simulink subsystem "Day3_Scenario_1"  (R2024a)
settings: Solver=VariableStepAuto  StartTime=0.0  StopTime=10.0  RelTol=1e-3
undefined symbols (not defined in the file): left_first_line_point_x, right_first_line_point_x
libraries: CarMaker4SL x6, slpidlib x1
settings Model: Creator=junhyung.cha  LastModifiedBy=hajin

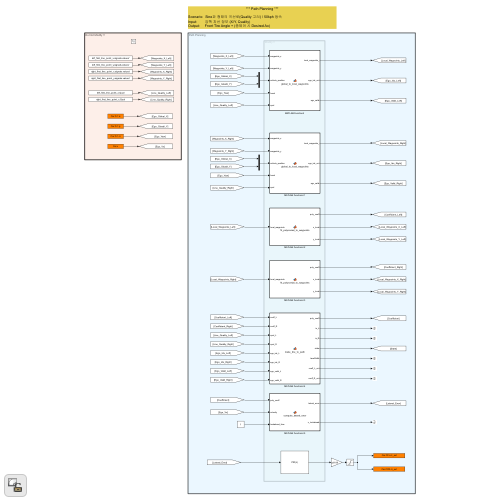
[thumbnail: Simulink's stored preview of the top-level diagram]
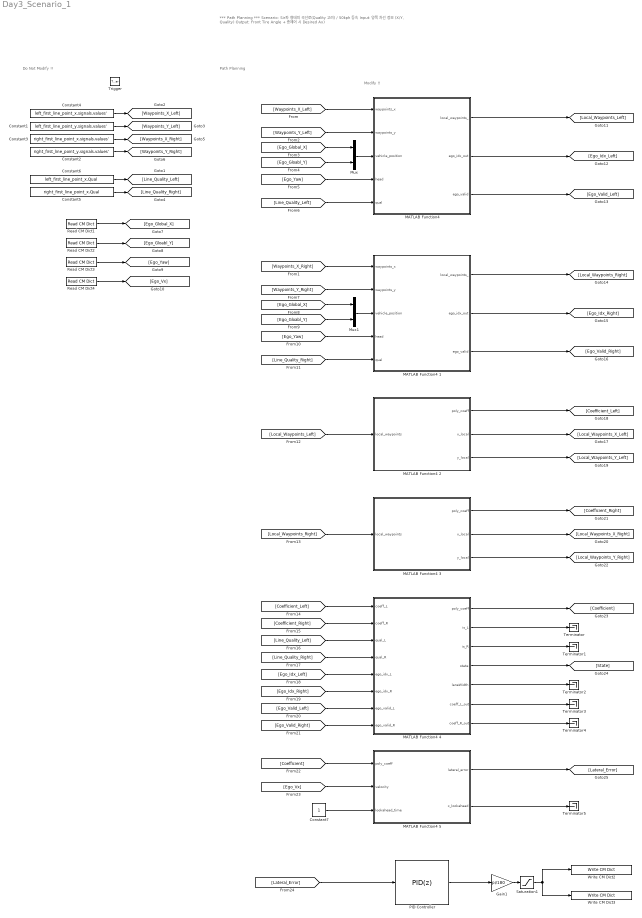
== system Day3_Scenario_1 ==
  note: Path Planning
  note: Do Not Modify !!
  note: Modify !!
  note: *** Path Planning ***
      |
      | Scenario: Sine파 형태의 곡선로(Quality 고려) / 50kph 등속
      | Input: 양쪽 차선 정보 (X/Y, Quality)
      | Output: Front Tire Angle + (종제어 시 Desired Ax)
  Trigger : TriggerPort  TriggerType=function-call  VariantControl=(inherit)
  Constant1 : Constant  Value=left_first_line_point_y.signals.values'
  Constant2 : Constant  Value=right_first_line_point_y.signals.values'
  Constant3 : Constant  Value=right_first_line_point_x.signals.values'
  Constant4 : Constant  Value=left_first_line_point_x.signals.values'
  Constant5 : Constant  Value=right_first_line_point_x.Qual
  Constant6 : Constant  Value=left_first_line_point_x.Qual
  Constant7 : Constant
  Gain1 : Gain  Gain=pi/180
  "MATLAB Function4 " : MATLAB Function  TreatAsAtomicUnit=on
  MATLAB Function4 1 : MATLAB Function  TreatAsAtomicUnit=on
  MATLAB Function4 2 : MATLAB Function  TreatAsAtomicUnit=on
  MATLAB Function4 3 : MATLAB Function  TreatAsAtomicUnit=on
  MATLAB Function4 4 : MATLAB Function  TreatAsAtomicUnit=on
  MATLAB Function4 5 : MATLAB Function  TreatAsAtomicUnit=on
  Mux : Mux  Inputs=2
  Mux1 : Mux  Inputs=2
  PID Controller : slpidlib/PID Controller  Controller=PID  Form=Parallel  TimeDomain=Discrete-time  UseExternalTs=off  SampleTime=-1  IntegratorMethod=Forward Euler  FilterMethod=Forward Euler  ControllerParametersSource=internal  P=3  I=0  UseKiTs=off  D=0.8  UseExternalDerivativeSource=off  N=100  UseFilter=on  TunerSelectOption=Transfer Function Based (PID Tuner App)  InitialConditionSource=internal  InitialConditionForIntegrator=0  InitialConditionForFilter=0  DifferentiatorICPrevScaledInput=0  ExternalReset=none  TrackingMode=off  Kt=1  LimitOutput=off  SatLimitsSource=internal  UpperSaturationLimit=inf  LowerSaturationLimit=-inf  LinearizeAsGain=on  AntiWindupMode=none  Kb=1  LimitIntegrator=off  UpperIntegratorSaturationLimit=inf  LowerIntegratorSaturationLimit=-inf  POutMin=[]  POutMax=[]  IOutMin=[]  IOutMax=[]  DOutMin=[]  DOutMax=[]  NOutMin=[]  NOutMax=[]  SumOutMin=[]  SumOutMax=[]  SaturationOutMin=[]  SaturationOutMax=[]  PParamMin=[]  PParamMax=[]  IParamMin=[]  IParamMax=[]  DParamMin=[]  DParamMax=[]  NParamMin=[]  NParamMax=[]  KbParamMin=[]  KbParamMax=[]  KtParamMin=[]  KtParamMax=[]  KbOutMin=[]  KbOutMax=[]  KtOutMin=[]  KtOutMax=[]  IntegratorOutMin=[]  IntegratorOutMax=[]  FilterOutMin=[]  FilterOutMax=[]  SumI1OutMin=[]  SumI1OutMax=[]  SumI2OutMin=[]  SumI2OutMax=[]  SumI3OutMin=[]  SumI3OutMax=[]  SumI4OutMin=[]  SumI4OutMax=[]  SumDOutMin=[]  SumDOutMax=[]  DifferentiatorOutMin=[]  DifferentiatorOutMax=[]  FilterDiffOutCoefMin=[]  FilterDiffOutCoefMax=[]  ReciprocalOutMin=[]  ReciprocalOutMax=[]  SumDenOutMin=[]  SumDenOutMax=[]  SumNumOutMin=[]  SumNumOutMax=[]  DivideOutMin=[]  DivideOutMax=[]  UdiffTsProdOutMin=[]  UdiffTsProdOutMax=[]  NTsProdOutMin=[]  NTsProdOutMax=[]  UintegralTsProdOutMin=[]  UintegralTsProdOutMax=[]  UngainTsProdOutMin=[]  UngainTsProdOutMax=[]  ClampingZeroOutDataTypeStr=Inherit: Inherit via back propagation  ClampingZeroOutMin=[]  ClampingZeroOutMax=[]  FilterDenConstantOutDataTypeStr=Inherit: Inherit via back propagation  FilterDenConstantOutMin=[]  FilterDenConstantOutMax=[]  PCopyOutDataTypeStr=Inherit: Inherit via back propagation  PCopyOutMin=[]  PCopyOutMax=[]  NCopyOutDataTypeStr=Inherit: Inherit via back propagation  NCopyOutMin=[]  NCopyOutMax=[]  IntegratorContinuousStateAttributes=''  IntegratorStateMustResolveToSignalObject=off  IntegratorRTWStateStorageClass=Auto  FilterContinuousStateAttributes=''  FilterStateMustResolveToSignalObject=off  FilterRTWStateStorageClass=Auto  ParallelPVariant=InternalParameters  IdealPVariant=Disabled  IVariant=InternalParameters  DVariant=InternalParameters  IntegratorVariant=Discrete  SatVariant=Disabled  AWVariant=Passthrough  PCopyVariant=Disabled  TRVariant=Disabled  FdbkBlocksVariant=Forward  IdealPFdbkVariant=Disabled  SatFdbkVariant=Disabled  DerivativeFilterVariant=ForwardEulerFilter  NVariant=InternalParameters  NCopyVariant=Disabled  FilterICVariant=InternalICsFilter  IntegratorICVariant=InternalICs  ExternalResetVariant=Disabled  TRSumVariant=Passthrough  SumFdbkVariant=Disabled  SumVariant=Sum_PID  TsampFilterVariant=InternalTs  TsampNgainVariant=Passthrough  TsampIntegralVariant=Disabled_SignalSpec  ExternalSaturationOutDataTypeStr=Inherit: Same as second input  DerivativeSourceVariant=ErrorSignal
  Read CM Dict1 : CarMaker4SL/Read CM Dict  xname=Car.Fr1.tx  xsync=off  xstime=Inherited
  Read CM Dict2 : CarMaker4SL/Read CM Dict  xname=Car.Fr1.ty  xsync=off  xstime=Inherited
  Read CM Dict3 : CarMaker4SL/Read CM Dict  xname=Car.Fr1.rz  xsync=off  xstime=Inherited
  Read CM Dict4 : CarMaker4SL/Read CM Dict  xname=Car.v  xsync=off  xstime=Inherited
  Saturation1 : Saturate  UpperLimit=2  LowerLimit=-2
  Terminator{,1..5} (6 alike) : Terminator
  Write CM Dict2 : CarMaker4SL/Write CM Dict  xname=Car.CFL.rz_ext  xsync=off
  Write CM Dict3 : CarMaker4SL/Write CM Dict  xname=Car.CFR.rz_ext  xsync=off
  wires:
  Constant4/1 -> [Waypoints_X_Left]
  Constant1/1 -> [Waypoints_Y_Left]
  Constant2/1 -> [Waypoints_Y_Right]
  Constant3/1 -> [Waypoints_X_Right]
  [Waypoints_X_Left] -> "MATLAB Function4 "/1(waypoints_x)
  [Waypoints_Y_Left] -> "MATLAB Function4 "/2(waypoints_y)
  Mux/1 -> "MATLAB Function4 "/3(vehicle_position)
  [Ego_Global_X] -> Mux/1
  Read CM Dict2/1 -> [Ego_Gloabl_Y]
  Read CM Dict1/1 -> [Ego_Global_X]
  [Ego_Gloabl_Y] -> Mux/2
  Read CM Dict3/1 -> [Ego_Yaw]
  [Ego_Yaw] -> "MATLAB Function4 "/4(head)
  Constant5/1 -> [Line_Quality_Right]
  Constant6/1 -> [Line_Quality_Left]
  [Line_Quality_Left] -> "MATLAB Function4 "/5(qual)
  [Line_Quality_Right] -> MATLAB Function4 1/5(qual)
  [Ego_Yaw] -> MATLAB Function4 1/4(head)
  [Ego_Gloabl_Y] -> Mux1/2
  [Ego_Global_X] -> Mux1/1
  [Waypoints_Y_Right] -> MATLAB Function4 1/2(waypoints_y)
  [Waypoints_X_Right] -> MATLAB Function4 1/1(waypoints_x)
  Mux1/1 -> MATLAB Function4 1/3(vehicle_position)
  "MATLAB Function4 "/3(ego_valid) -> [Ego_Valid_Left]
  "MATLAB Function4 "/2(ego_idx_out) -> [Ego_Idx_Left]
  "MATLAB Function4 "/1(local_waypoints_) -> [Local_Waypoints_Left]
  MATLAB Function4 1/1(local_waypoints_) -> [Local_Waypoints_Right]
  MATLAB Function4 1/2(ego_idx_out) -> [Ego_Idx_Right]
  MATLAB Function4 1/3(ego_valid) -> [Ego_Valid_Right]
  [Local_Waypoints_Left] -> MATLAB Function4 2/1(local_waypoints)
  [Local_Waypoints_Right] -> MATLAB Function4 3/1(local_waypoints)
  MATLAB Function4 2/1(poly_coeff) -> [Coefficient_Left]
  MATLAB Function4 2/2(x_local) -> [Local_Waypoints_X_Left]
  MATLAB Function4 2/3(y_local) -> [Local_Waypoints_Y_Left]
  MATLAB Function4 3/3(y_local) -> [Local_Waypoints_Y_Right]
  MATLAB Function4 3/2(x_local) -> [Local_Waypoints_X_Right]
  MATLAB Function4 3/1(poly_coeff) -> [Coefficient_Right]
  [Coefficient_Left] -> MATLAB Function4 4/1(coeff_L)
  [Coefficient_Right] -> MATLAB Function4 4/2(coeff_R)
  [Line_Quality_Left] -> MATLAB Function4 4/3(qual_L)
  [Line_Quality_Right] -> MATLAB Function4 4/4(qual_R)
  [Ego_Idx_Left] -> MATLAB Function4 4/5(ego_idx_L)
  [Ego_Idx_Right] -> MATLAB Function4 4/6(ego_idx_R)
  [Ego_Valid_Left] -> MATLAB Function4 4/7(ego_valid_L)
  [Ego_Valid_Right] -> MATLAB Function4 4/8(ego_valid_R)
  MATLAB Function4 4/1(poly_coeff) -> [Coefficient]
  MATLAB Function4 4/4(state) -> [State]
  MATLAB Function4 4/2(is_L) -> Terminator/1
  MATLAB Function4 4/3(is_R) -> Terminator1/1
  MATLAB Function4 4/6(coeff_L_out) -> Terminator3/1
  MATLAB Function4 4/5(laneWidth) -> Terminator2/1
  MATLAB Function4 4/7(coeff_R_out) -> Terminator4/1
  [Coefficient] -> MATLAB Function4 5/1(poly_coeff)
  Read CM Dict4/1 -> [Ego_Vx]
  [Ego_Vx] -> MATLAB Function4 5/2(velocity)
  Constant7/1 -> MATLAB Function4 5/3(lookahead_time)
  Saturation1/1 -> Write CM Dict3/1, Write CM Dict2/1
  Gain1/1 -> Saturation1/1
  MATLAB Function4 5/1(lateral_error) -> [Lateral_Error]
  MATLAB Function4 5/2(x_lookahead) -> Terminator5/1
  [Lateral_Error] -> PID Controller/1
  PID Controller/1 -> Gain1/1

== matlab function Day3_Scenario_1/MATLAB Function4  ==
  settings: sampleTime=0.1
  data: waypoints_x input; waypoints_y input; local_waypoints_ output; vehicle_position input; head input; qual input; ego_idx_out output; ego_valid output
function [local_waypoints_, ego_idx_out, ego_valid] = global_to_local_waypoints(waypoints_x, waypoints_y, vehicle_position, head, qual)
% 전역 좌표계 waypoint를 ego 차량 기준 local 좌표계로 변환하는 함수
%
% 입력:
%   waypoints_x       : 전역 waypoint X 좌표 배열
%   waypoints_y       : 전역 waypoint Y 좌표 배열
%   vehicle_position  : ego 차량 위치 [X, Y]
%   head              : ego 차량 yaw angle [rad]
%   qual              : 차선 quality 값
%
% 출력:
%   local_waypoints_  : ego 기준 local waypoint [x_local, y_local]
%   ego_idx_out       : ego 앞쪽에서 처음으로 유효한 waypoint의 원본 index
%   ego_valid         : 경로 생성에 사용할 수 있는 waypoint가 충분한지 여부

% waypoint 개수
N = length(waypoints_x);

% 출력 초기화
% NaN으로 채워두면 유효하지 않은 점은 이후 polyfit에서 제외하기 쉬움
local_waypoints_ = NaN(N, 2);
ego_idx_out = 0;
ego_valid = false;

% ego 차량의 전역 위치
ego_x = vehicle_position(1);
ego_y = vehicle_position(2);

% yaw 회전 변환을 위한 값
c = cos(head);
s = sin(head);

% 유효한 local waypoint 개수
valid_count = 0;

% 전방 첫 번째 유효 waypoint의 원본 index 저장용
first_valid_idx = 0;

for i = 1:N

    % quality가 scalar로 들어오는 경우와 배열로 들어오는 경우 모두 처리
    if length(qual) == 1
        point_valid = qual > 0.5;
    else
        point_valid = qual(i) > 0.5;
    end

    % quality가 유효한 점만 사용
    if point_valid

        % ego 위치 기준으로 평행이동
        dx = waypoints_x(i) - ego_x;
        dy = waypoints_y(i) - ego_y;

        % global 좌표계에서 local 좌표계로 회전 변환
        % ego 차량 진행 방향이 local x축
        x_local =  c * dx + s * dy;
        y_local = -s * dx + c * dy;

        % 차량 앞쪽에 있는 waypoint만 사용
        if x_local >= 0
            valid_count = valid_count + 1;

            local_waypoints_(valid_count, 1) = x_local;
            local_waypoints_(valid_count, 2) = y_local;

            % 처음 발견한 전방 유효 waypoint index 저장
            if first_valid_idx == 0
                first_valid_idx = i;
            end
        end
    end
end

% ego 앞쪽에서 처음으로 유효한 waypoint의 원본 index
ego_idx_out = first_valid_idx;

% 3차 다항식 피팅을 하려면 최소 4개의 점이 필요
if valid_count >= 4
    ego_valid = true;
else
    ego_valid = false;
end

end

== matlab function Day3_Scenario_1/MATLAB Function4 1 ==
  settings: sampleTime=0.1
  data: waypoints_x input; waypoints_y input; local_waypoints_ output; vehicle_position input; head input; qual input; ego_idx_out output; ego_valid output
function [local_waypoints_, ego_idx_out, ego_valid] = global_to_local_waypoints(waypoints_x, waypoints_y, vehicle_position, head, qual)
% 전역 좌표계의 waypoint를 ego 차량 기준 local 좌표계로 변환하는 함수
%
% 입력:
%   waypoints_x      : 전역 좌표계 waypoint X 배열
%   waypoints_y      : 전역 좌표계 waypoint Y 배열
%   vehicle_position : ego 차량의 전역 위치 [X, Y]
%   head             : ego 차량의 yaw angle [rad]
%   qual             : 차선 품질 값
%
% 출력:
%   local_waypoints_ : ego 기준 local waypoint [x_local, y_local]
%   ego_idx_out      : ego 앞쪽에서 처음 발견된 유효 waypoint index
%   ego_valid        : 경로 생성에 사용할 수 있는 waypoint가 충분한지 여부

% 입력 waypoint를 column vector로 변환
waypoints_x = waypoints_x(:);
waypoints_y = waypoints_y(:);

% waypoint 개수 확인
N = length(waypoints_x);

% 출력 초기화
% 유효하지 않은 waypoint는 NaN으로 남김
local_waypoints_ = NaN(N, 2);
ego_idx_out = 0;
ego_valid = false;

% ego 차량의 전역 위치
ego_x = vehicle_position(1);
ego_y = vehicle_position(2);

% heading angle에 대한 삼각함수 계산
c = cos(head);
s = sin(head);

% 유효한 전방 waypoint 개수
valid_count = 0;

% quality 기준값
quality_threshold = 0.5;

for i = 1:N

    % quality가 scalar로 들어오는 경우
    if length(qual) == 1
        point_valid = qual > quality_threshold;

    % quality가 waypoint별 배열로 들어오는 경우
    else
        point_valid = qual(i) > quality_threshold;
    end

    % quality가 좋지 않으면 해당 waypoint는 사용하지 않음
    if point_valid

        % ego 차량 위치 기준으로 평행 이동
        dx = waypoints_x(i) - ego_x;
        dy = waypoints_y(i) - ego_y;

        % global 좌표계에서 ego 기준 local 좌표계로 회전 변환
        % local x축 : 차량 진행 방향
        % local y축 : 차량 좌측 방향
        x_local =  c * dx + s * dy;
        y_local = -s * dx + c * dy;

        % 차량 앞쪽에 있는 waypoint만 사용
        if x_local >= 0

            valid_count = valid_count + 1;

            % local waypoint 저장
            local_waypoints_(valid_count, 1) = x_local;
            local_waypoints_(valid_count, 2) = y_local;

            % ego 앞쪽에서 처음 발견된 waypoint의 원본 index 저장
            if ego_idx_out == 0
                ego_idx_out = i;
            end
        end
    end
end

% 3차 다항식 fitting을 위해서는 최소 4개의 점이 필요
if valid_count >= 4
    ego_valid = true;
else
    ego_valid = false;
end

end

== matlab function Day3_Scenario_1/MATLAB Function4 2 ==
  settings: sampleTime=0.1
  data: local_waypoints input; poly_coeff output; x_local output; y_local output
function [poly_coeff, x_local, y_local] = fit_polynomial_to_waypoints(local_waypoints)
% local waypoint들을 이용해 3차 다항식 계수를 계산하는 함수
% Simulink MATLAB Function 블록에서 가변 크기 오류를 피하기 위한 고정 크기 코드

% 입력 waypoint 개수
N = size(local_waypoints, 1);

% 출력 초기화
% poly_coeff는 항상 [4x1] 고정
poly_coeff = zeros(4, 1);

% x_local, y_local은 입력 waypoint 개수만큼 고정
x_local = zeros(N, 1);
y_local = zeros(N, 1);

% 다항식 피팅에 사용할 최대 점 개수
% 너무 많은 점을 모두 쓰지 않고 앞쪽 유효 점 일부만 사용
max_fit_num = 20;

% 피팅용 배열 고정 크기 선언
x_fit = zeros(max_fit_num, 1);
y_fit = zeros(max_fit_num, 1);

valid_count = 0;

% 유효한 waypoint 수집
for i = 1:N
    x = local_waypoints(i, 1);
    y = local_waypoints(i, 2);

    % NaN이 아니고 차량 앞쪽에 있는 점만 사용
    if isfinite(x) && isfinite(y) && x >= 0

        % 출력 확인용 local 좌표 저장
        x_local(i) = x;
        y_local(i) = y;

        % 피팅에는 최대 max_fit_num개만 사용
        if valid_count < max_fit_num
            valid_count = valid_count + 1;
            x_fit(valid_count) = x;
            y_fit(valid_count) = y;
        end
    end
end

% 유효한 점이 4개 이상이면 3차 다항식 피팅
if valid_count >= 4

    % 고정 크기 행렬 사용
    A = zeros(max_fit_num, 4);
    b = zeros(max_fit_num, 1);

    for i = 1:max_fit_num
        x = x_fit(i);

        A(i, 1) = x^3;
        A(i, 2) = x^2;
        A(i, 3) = x;
        A(i, 4) = 1;

        b(i) = y_fit(i);
    end

    % 최소자승법
    % 결과는 항상 [4x1]
    coeff_temp = A \ b;

    poly_coeff(1) = coeff_temp(1);
    poly_coeff(2) = coeff_temp(2);
    poly_coeff(3) = coeff_temp(3);
    poly_coeff(4) = coeff_temp(4);

% 유효한 점이 2~3개면 1차 직선으로 대체
elseif valid_count >= 2

    A_line = zeros(max_fit_num, 2);
    b_line = zeros(max_fit_num, 1);

    for i = 1:max_fit_num
        x = x_fit(i);

        A_line(i, 1) = x;
        A_line(i, 2) = 1;

        b_line(i) = y_fit(i);
    end

    line_coeff = A_line \ b_line;

    % 3차 계수 형태로 고정 출력
    % y = 0*x^3 + 0*x^2 + m*x + b
    poly_coeff(1) = 0;
    poly_coeff(2) = 0;
    poly_coeff(3) = line_coeff(1);
    poly_coeff(4) = line_coeff(2);

else

    % 유효한 점이 부족하면 직진 경로
    poly_coeff(1) = 0;
    poly_coeff(2) = 0;
    poly_coeff(3) = 0;
    poly_coeff(4) = 0;

end

end

== matlab function Day3_Scenario_1/MATLAB Function4 3 ==
  settings: sampleTime=0.1
  data: local_waypoints input; poly_coeff output size=[4 1]; x_local output; y_local output
function [poly_coeff, x_local, y_local] = fit_polynomial_to_waypoints(local_waypoints)
% local waypoint들을 이용해 3차 다항식 계수를 계산하는 함수
%
% 입력:
%   local_waypoints : ego 차량 기준 local waypoint
%                     각 행은 [x_local, y_local]
%
% 출력:
%   poly_coeff : 3차 다항식 계수
%                y = a*x^3 + b*x^2 + c*x + d
%                [a; b; c; d] 형태
%   x_local    : 유효한 local x 좌표
%   y_local    : 유효한 local y 좌표

% waypoint 개수 확인
N = size(local_waypoints, 1);

% 출력 초기화
poly_coeff = zeros(4, 1);
x_local = zeros(N, 1);
y_local = zeros(N, 1);

% 유효한 waypoint 개수
valid_count = 0;

% 유효한 waypoint만 따로 저장
x_valid = zeros(N, 1);
y_valid = zeros(N, 1);

for i = 1:N

    x = local_waypoints(i, 1);
    y = local_waypoints(i, 2);

    % NaN이 아니고 차량 앞쪽에 있는 waypoint만 사용
    if isfinite(x) && isfinite(y) && x >= 0

        valid_count = valid_count + 1;

        x_valid(valid_count) = x;
        y_valid(valid_count) = y;

        x_local(valid_count) = x;
        y_local(valid_count) = y;
    end
end

% 유효한 점이 4개 이상이면 3차 다항식 피팅
if valid_count >= 4

    % 최소자승법을 위한 행렬 생성
    % y = a*x^3 + b*x^2 + c*x + d
    A = zeros(valid_count, 4);
    b = zeros(valid_count, 1);

    for i = 1:valid_count
        x = x_valid(i);

        A(i, 1) = x^3;
        A(i, 2) = x^2;
        A(i, 3) = x;
        A(i, 4) = 1;

        b(i) = y_valid(i);
    end

    % 최소자승법으로 다항식 계수 계산
    % poly_coeff = [a; b; c; d]
    poly_coeff = A \ b;

% 유효한 점이 2개 이상이면 1차 직선으로 대체
elseif valid_count >= 2

    % y = m*x + b 형태로 피팅
    A = zeros(valid_count, 2);
    b = zeros(valid_count, 1);

    for i = 1:valid_count
        x = x_valid(i);

        A(i, 1) = x;
        A(i, 2) = 1;

        b(i) = y_valid(i);
    end

    line_coeff = A \ b;

    % 3차 계수 형식으로 변환
    % y = 0*x^3 + 0*x^2 + m*x + b
    poly_coeff = [0; 0; line_coeff(1); line_coeff(2)];

else

    % 유효한 점이 부족하면 직진 경로로 처리
    poly_coeff = [0; 0; 0; 0];

end

end

== matlab function Day3_Scenario_1/MATLAB Function4 4 ==
  settings: sampleTime=0.1
  data: coeff_L input; poly_coeff output; is_L output; is_R output; coeff_R input; qual_L input; qual_R input; ego_idx_L input; ego_idx_R input; ego_valid_L input; ego_valid_R input; state output; laneWidth output; coeff_L_out output; coeff_R_out output
function [poly_coeff,is_L,is_R,state,laneWidth,coeff_L_out,coeff_R_out] = make_line_to_path(coeff_L,coeff_R,qual_L,qual_R,ego_idx_L, ego_idx_R,ego_valid_L,ego_valid_R)
% 좌/우 차선 계수를 이용해 중앙 주행 경로를 생성하는 함수
%
% poly_coeff는 항상 [4x1] 고정 크기
% y = a*x^3 + b*x^2 + c*x + d

persistent laneWidth_mem prev_poly firstRun

% 처음 실행될 때 초기화
if isempty(firstRun)
    laneWidth_mem = 4.0;        % 초기 차선폭 [m]
    prev_poly = zeros(4, 1);    % 이전 경로 계수 [4x1]
    firstRun = 1;
end

% 출력 크기 고정
poly_coeff = zeros(4, 1);
coeff_L_out = zeros(4, 1);
coeff_R_out = zeros(4, 1);

is_L = 0;
is_R = 0;
state = 0;
laneWidth = laneWidth_mem;

% 입력 차선 계수를 고정 크기 변수로 복사
cL = zeros(4, 1);
cR = zeros(4, 1);

for i = 1:4
    cL(i) = coeff_L(i);
    cR(i) = coeff_R(i);
end

% 차선 품질 기준값
quality_threshold = 0.5;

% qual_L, qual_R이 벡터로 들어올 수 있으므로 scalar logical로 변환
qual_L_ok = any(qual_L(:) > quality_threshold);
qual_R_ok = any(qual_R(:) > quality_threshold);

% ego index와 valid도 scalar로 사용
ego_idx_L_s = ego_idx_L(1);
ego_idx_R_s = ego_idx_R(1);

ego_valid_L_s = ego_valid_L(1);
ego_valid_R_s = ego_valid_R(1);

% 왼쪽 / 오른쪽 차선 유효 여부 판단
left_valid = qual_L_ok && (ego_valid_L_s > 0) && (ego_idx_L_s > 0);
right_valid = qual_R_ok && (ego_valid_R_s > 0) && (ego_idx_R_s > 0);

% 계수에 NaN 또는 Inf가 있는지 확인
coeff_L_ok = true;
coeff_R_ok = true;

for i = 1:4
    if ~isfinite(cL(i))
        coeff_L_ok = false;
    end

    if ~isfinite(cR(i))
        coeff_R_ok = false;
    end
end

left_valid = left_valid && coeff_L_ok;
right_valid = right_valid && coeff_R_ok;

% ===============================
% 1. 양쪽 차선이 모두 유효한 경우
% ===============================
if left_valid && right_valid

    % 좌우 차선 평균으로 중앙 경로 생성
    poly_coeff = (cL + cR) / 2.0;

    % 차선폭 갱신
    % 마지막 계수는 y절편이므로 좌우 y절편 차이를 차선폭으로 사용
    laneWidth_mem = abs(cL(4) - cR(4));

    coeff_L_out = cL;
    coeff_R_out = cR;

    is_L = 1;
    is_R = 1;
    state = 2;

% ===============================
% 2. 왼쪽 차선만 유효한 경우
% ===============================
elseif left_valid && ~right_valid

    % 왼쪽 차선에서 오른쪽으로 차선폭 절반 이동
    poly_coeff = cL;
    poly_coeff(4) = poly_coeff(4) - laneWidth_mem / 2.0;

    % 오른쪽 가상 차선 생성
    coeff_L_out = cL;
    coeff_R_out = cL;
    coeff_R_out(4) = coeff_R_out(4) - laneWidth_mem;

    is_L = 1;
    is_R = 0;
    state = 1;

% ===============================
% 3. 오른쪽 차선만 유효한 경우
% ===============================
elseif ~left_valid && right_valid

    % 오른쪽 차선에서 왼쪽으로 차선폭 절반 이동
    poly_coeff = cR;
    poly_coeff(4) = poly_coeff(4) + laneWidth_mem / 2.0;

    % 왼쪽 가상 차선 생성
    coeff_R_out = cR;
    coeff_L_out = cR;
    coeff_L_out(4) = coeff_L_out(4) + laneWidth_mem;

    is_L = 0;
    is_R = 1;
    state = -1;

% ===============================
% 4. 양쪽 차선이 모두 유효하지 않은 경우
% ===============================
else

    % 둘 다 안 보이면 이전 경로 유지
    poly_coeff = prev_poly;

    coeff_L_out = zeros(4, 1);
    coeff_R_out = zeros(4, 1);

    is_L = 0;
    is_R = 0;
    state = 0;

end

% 차선폭 출력
laneWidth = laneWidth_mem;

% 다음 step을 위해 현재 경로 저장
prev_poly = poly_coeff;

end

== matlab function Day3_Scenario_1/MATLAB Function4 5 ==
  settings: sampleTime=0.1
  data: poly_coeff input; lateral_error output; x_lookahead output; velocity input; lookahead_time input
function [lateral_error, x_lookahead] = compute_lateral_error(poly_coeff, velocity, lookahead_time)
% 다항식 경로에서 lookahead 지점의 횡방향 오차를 계산하는 함수
%
% 입력:
%   poly_coeff     : 경로 다항식 계수 [a; b; c; d]
%                    y = a*x^3 + b*x^2 + c*x + d
%   velocity       : ego 차량 속도 [m/s]
%   lookahead_time : 전방 주시 시간 [s]
%
% 출력:
%   lateral_error  : lookahead 지점에서의 횡방향 오차 [m]
%   x_lookahead    : 전방 주시 거리 [m]

% 전방 주시 거리 계산
% 속도가 빠를수록 더 먼 지점을 바라봄
x_lookahead = velocity * lookahead_time;

% lookahead 거리가 너무 작아지는 것을 방지
if x_lookahead < 0.5
    x_lookahead = 0.5;
end

% lookahead 거리가 너무 커지는 것을 방지
if x_lookahead > 20.0
    x_lookahead = 20.0;
end

% 다항식 계수 분리
a = poly_coeff(1);
b = poly_coeff(2);
c = poly_coeff(3);
d = poly_coeff(4);

% lookahead 지점에서의 경로 y값 계산
% y = a*x^3 + b*x^2 + c*x + d
y_lookahead = a * x_lookahead^3 + ...
              b * x_lookahead^2 + ...
              c * x_lookahead + ...
              d;

% ego 차량은 local 좌표계에서 y = 0에 있다고 보기 때문에
% 경로의 y값이 곧 횡방향 오차가 됨
lateral_error = y_lookahead;

end
